simulink model "tank"  (Simulink 4.00)
settings: Solver=ode45  StartTime=0.0  StopTime=10.0  RelTol=1e-3
settings Model: LastModifiedBy=hespanha  BlockReductionOpt=off

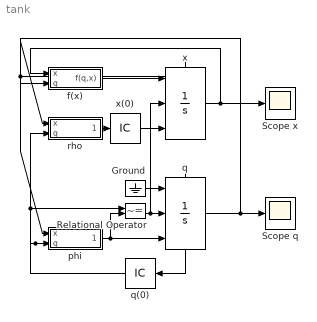
== system tank ==
  Ground : Ground
  Relational Operator : RelationalOperator  Operator=~=
  Scope q : Scope
      settings: TimeRange=10  YMin=0  YMax=5  SaveToWorkspace=off  LimitDataPoints=on  MaxDataPoints=5000
  Scope x : Scope
      settings: TimeRange=10  YMin=-1  YMax=5  SaveToWorkspace=off  SaveName=ScopeData  LimitDataPoints=on  MaxDataPoints=5000
  f(x) : Subsystem  Description=f(x)
      settings: RTWFcnNameOpts=Auto  RTWFileNameOpts=Auto
  phi : Subsystem  Description=f(x)
      settings: RTWFcnNameOpts=Auto  RTWFileNameOpts=Auto
  q : Integrator  ExternalReset=rising  InitialConditionSource=external  InitialCondition=0  LimitOutput=off  UpperSaturationLimit=inf  LowerSaturationLimit=-inf  ShowSaturationPort=off  ShowStatePort=on  AbsoluteTolerance=auto
  q(0) : InitialCondition  Orientation=left  Value=1
  rho : Subsystem  Description=f(x)
      settings: RTWFcnNameOpts=Auto  RTWFileNameOpts=Auto
  x : Integrator  ExternalReset=rising  InitialConditionSource=external  InitialCondition=0  LimitOutput=off  UpperSaturationLimit=inf  LowerSaturationLimit=-inf  ShowSaturationPort=off  ShowStatePort=on  AbsoluteTolerance=auto
  x(0) : InitialCondition  Value=[4;0]
  wires:
  x(0)/1 -> x/3
  f(x)/1(f(q,x)) -> x/1
  x/1 -> Scope x/1, f(x)/1(x)
  q/1 -> Scope q/1, f(x)/2(q)
  Ground/1 -> q/1
  Relational Operator/1 -> q/2, x/2
  phi/1(phi(q,x)) -> Relational Operator/2, q/3
  q/State -> q(0)/1
  x/State -> phi/1(x), rho/1(x)
  rho/1(rho(q,x)) -> x(0)/1
  q(0)/1 -> phi/2(q), rho/2(q), Relational Operator/1

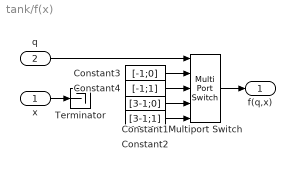
== system tank/f(x) ==
  x : Inport  Port=1
  q : Inport  Port=2
  Constant1 : Constant  Value=[3-1;0]
  Constant2 : Constant  Value=[3-1;1]
  Constant3 : Constant  Value=[-1;0]
  Constant4 : Constant  Value=[-1;1]
  Multiport Switch : MultiPortSwitch  Inputs=4
  Terminator : Terminator
  f(q,x) : Outport  Port=1
  wires:
  q/1 -> Multiport Switch/1
  Constant3/1 -> Multiport Switch/2
  Multiport Switch/1 -> f(q,x)/1
  Constant4/1 -> Multiport Switch/3
  Constant1/1 -> Multiport Switch/4
  Constant2/1 -> Multiport Switch/5
  x/1 -> Terminator/1

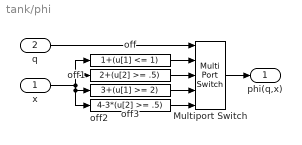
== system tank/phi ==
  x : Inport  Port=1
  q : Inport  Port=2
  Multiport Switch : MultiPortSwitch  Inputs=4
  off : Fcn  Expr=1+(u[1] <= 1)
  off1 : Fcn  Expr=2+(u[2] >= .5)
  off2 : Fcn  Expr=4-3*(u[2] >= .5)
  off3 : Fcn  Expr=3+(u[1] >= 2)
  phi(q,x) : Outport  Port=1
  wires:
  q/1 -> Multiport Switch/1
  Multiport Switch/1 -> phi(q,x)/1
  off/1 -> Multiport Switch/2
  off1/1 -> Multiport Switch/3
  off3/1 -> Multiport Switch/4
  x/1 -> off/1, off1/1, off3/1, off2/1
  off2/1 -> Multiport Switch/5

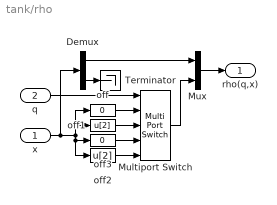
== system tank/rho ==
  x : Inport  Port=1
  q : Inport  Port=2
  Demux : Demux  Outputs=2  BusSelectionMode=off
  Multiport Switch : MultiPortSwitch  Inputs=4
  Mux : Mux  Inputs=2
  Terminator : Terminator
  off : Fcn  Expr=0
  off1 : Fcn  Expr=u[2]
  off2 : Fcn  Expr=u[2]
  off3 : Fcn  Expr=0
  rho(q,x) : Outport  Port=1
  wires:
  off2/1 -> Multiport Switch/5
  x/1 -> off2/1, off3/1, off1/1, off/1, Demux/1
  off3/1 -> Multiport Switch/4
  off1/1 -> Multiport Switch/3
  off/1 -> Multiport Switch/2
  q/1 -> Multiport Switch/1
  Mux/1 -> rho(q,x)/1
  Demux/1 -> Mux/1
  Multiport Switch/1 -> Mux/2
  Demux/2 -> Terminator/1
